simulink model "SIL_PIL_extern"  (R2023b)
settings: Solver=FixedStepDiscrete  StartTime=0.0  StopTime=10.0  FixedStep=Ts  RelTol=1e-3  EnableMultiTasking=on
values from neighbouring files (symbols this model uses):
  Ts = 0.005    [attempt.m]    (also in model_approximation.m; tuning.m)
undefined symbols (not defined in the file or in its folder): sys_discrete_motor
settings Model: CodeVerificationMode=processor-in-the-loop (pil)  ExtModeTrigDuration=10  Creator=giova  LastModifiedBy=david
settings OptimizationCC: EnhancedBackFolding=on  PassReuseOutputArgsAs=Individual arguments  ZeroExternalMemoryAtStartup=off  ZeroInternalMemoryAtStartup=off  MaxStackSize=64  OptimizeBlockOrder=speed  DifferentSizesBufferReuse=on  OptimizationCustomize=off  EfficientTunableParamExpr=on
settings DebuggingCC: ParameterTunabilityLossMsg=error
settings HardwareCC: ProdBitPerPointer=32  ProdBitPerSizeT=32  ProdBitPerPtrDiffT=32  ProdLargestAtomicInteger=Long  ProdLargestAtomicFloat=Double  ProdWordSize=32  ProdLongLongMode=on  ProdHWDeviceType=ARM Compatible->ARM Cortex
settings SFSimCC: MATLABDynamicMemAlloc=off
settings RTWCC: Description=Embedded Coder  SystemTargetFile=ert.tlc  HardwareBoard=STM32 Nucleo F401RE  TemplateMakefile=ert_default_tmf  Toolchain=GNU Tools for ARM Embedded Processors  PortableWordSizes=on
settings CodeAppCC: ForceParamTrailComments=on  IgnoreCustomStorageClasses=off  OperatorAnnotations=on  SimulinkDataObjDesc=on  SFDataObjDesc=on  InsertBlockDesc=on
settings ERTTargetCC: ExtModeTransport=3  ExtModeStaticAlloc=on  ExtModeStaticAllocSize=2000  ExtModeMexFile=ext_xcp  ExtModeIntrfLevel=Level2 - Open

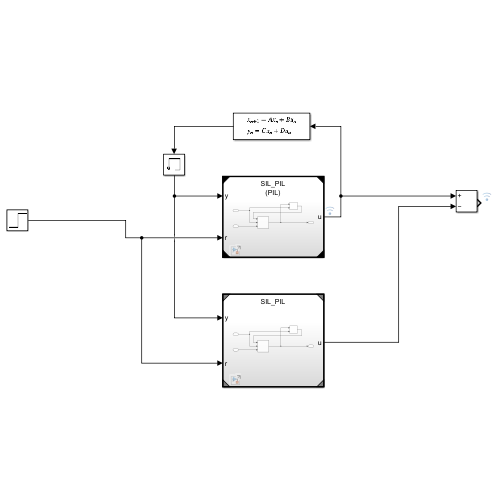
[thumbnail: Simulink's stored preview of the top-level diagram]
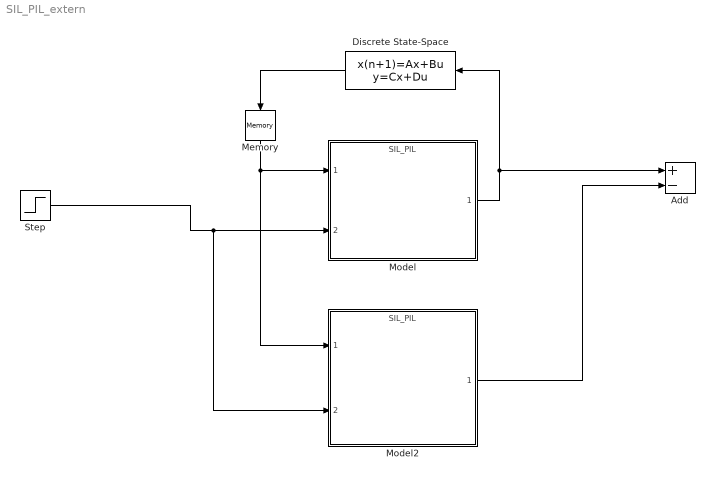
== system SIL_PIL_extern ==
  Add : Sum  Inputs=+-
  Discrete State-Space : DiscreteStateSpace  A=sys_discrete_motor.A  B=sys_discrete_motor.B  C=sys_discrete_motor.C  D=sys_discrete_motor.D  InitialCondition=[0 0 0]  SampleTime=Ts
  Memory : Memory
  Model : ModelReference  ModelNameDialog=SIL_PIL.slx  SimulationMode=Processor-in-the-loop (PIL)  ModelReferenceVersion=1.10
  Model2 : ModelReference  ModelNameDialog=SIL_PIL.slx  SimulationMode=Normal  ModelReferenceVersion=1.10
  Step : Step  Time=0  After=3.14
  wires:
  Step/1 -> Model2/2, Model/2
  Discrete State-Space/1 -> Memory/1
  Model2/1 -> Add/2
  Model/1 -> Discrete State-Space/1, Add/1
  Memory/1 -> Model2/1, Model/1
